simulink model "Single_Phase_grid-connected-inverter_Droop_inverter2"  (R2016b)
settings: Solver=VariableStepAuto  StartTime=0.0  StopTime=30  RelTol=1e-3
libraries: spsAlphaBetaZerotodq0Lib x4, simulink x4, spsSeriesRLCBranchLib x3, spsCurrentMeasurementLib x2, spsPWMGenerator2LevelLib x1, spsdq0toAlphaBetaZeroLib x1, spsDCVoltageSourceLib x1, spsPowerLib x1, spsUniversalBridgeLib x1, spsVoltageMeasurementLib x1, spspowerguiLib x1
settings Model: Creator=SALLEY  LastModifiedBy=49916
settings SimscapeCC: SimscapeNormalizeSystem=off

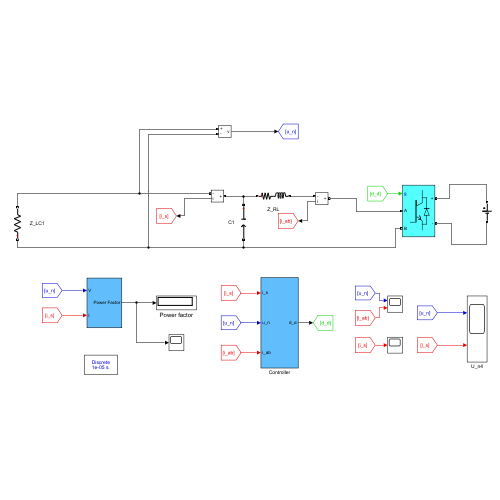
[thumbnail: Simulink's stored preview of the top-level diagram]
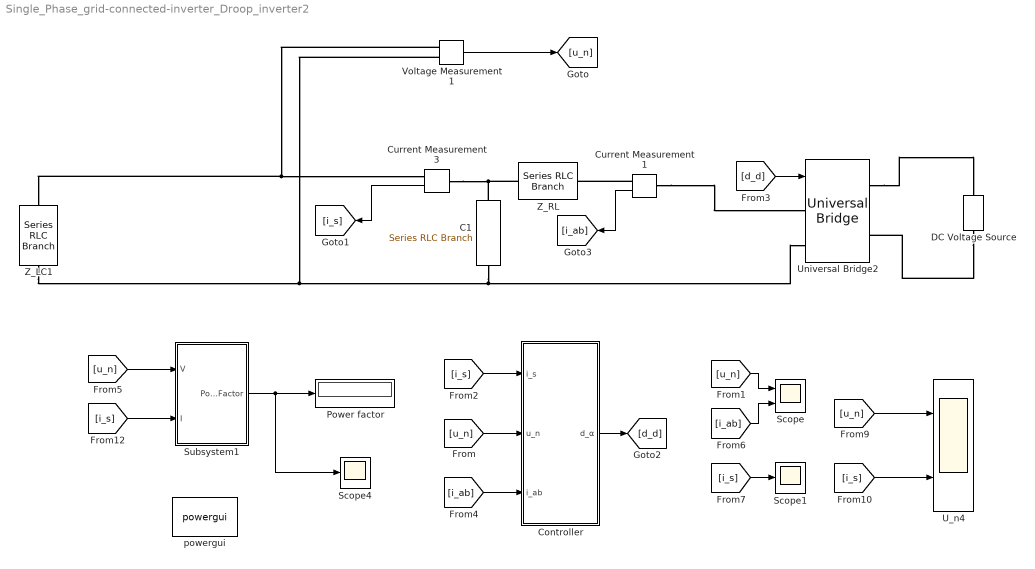
== system Single_Phase_grid-connected-inverter_Droop_inverter2 ==
  C1 : spsSeriesRLCBranchLib/Series RLC Branch  LConnTagsString=__new0  RConnTagsString=__new0  BranchType=C  Resistance=1  Inductance=1e-3  SetiL0=off  InitialCurrent=0  Capacitance=2e-5  Setx0=off  InitialVoltage=1500  Measurements=None
  Controller : Subsystem
  Current Measurement1 : spsCurrentMeasurementLib/Current Measurement  PhasorSimulation=off  OutputType=Complex  PSBequivalent=0
  Current Measurement3 : spsCurrentMeasurementLib/Current Measurement  PhasorSimulation=off  OutputType=Complex  PSBequivalent=0
  DC Voltage Source : spsDCVoltageSourceLib/DC Voltage Source  Amplitude=800  Measurements=None
  Power factor : Display
  Scope : Scope  NumInputPorts=2
  Scope1 : Scope
  Scope4 : Scope
  Subsystem1 : Subsystem
  U_n4 : Scope  NumInputPorts=2
  Universal Bridge2 : spsUniversalBridgeLib/Universal Bridge  Arms=2  SnubberResistance=1e5  SnubberCapacitance=inf  Device=IGBT / Diodes  Ron=1e-3  Lon=0  ForwardVoltages="[  0  0  ]"  ForwardVoltage=0  GTOparameters=[ 10e-6 , 20e-6 ]  IGBTparameters=[ 1e-6 , 2e-6 ]  Measurements=None  Measurements_2=None  converterType=Rectifier
  Voltage Measurement1 : spsVoltageMeasurementLib/Voltage Measurement  PhasorSimulation=off  OutputType=Complex  PSBequivalent=0
  Z_LC1 : spsSeriesRLCBranchLib/Series RLC Branch  LConnTagsString=__new0  RConnTagsString=__new0  BranchType=R  Resistance=2  Inductance=0  SetiL0=off  InitialCurrent=400  Capacitance=9.85e-3  Setx0=off  InitialVoltage=0  Measurements=None
  Z_RL : spsSeriesRLCBranchLib/Series RLC Branch  LConnTagsString=__new0  RConnTagsString=__new0  BranchType=RL  Resistance=0.2  Inductance=3e-3  SetiL0=off  InitialCurrent=400  Capacitance=9.85e-3  Setx0=off  InitialVoltage=0  Measurements=None
  powergui : spspowerguiLib/powergui  Priority=1  SimulationMode=Discrete  SampleTime=10e-6  frequency=60  Iterations=50  frequencyindice=0  Pbase=100e6  ErrMax=1e-4  UnitsV=kV  UnitsW=MW  buscounter=0  FunctionMessages=off  echomessages=off  EnableUseOfTLC=off  CurrentSourceSwitches=off  DisableSnubberDevices=off  DisableRonSwitches=off  DisableVfSwitches=off  DisplayEquations=off  AutomaticDiscreteSolvers=off  SolverType=Tustin/Backward Euler (TBE)  Interpol=off  ExternalGateDelay=off  methode=off  Ts=10  x0status=blocks  SPID=off  SwTol=0  HookPort=off  NonlinearTolerance=1e-4  nMaxIteration=100  ContinueOnMaxIteration=off  RestoreLinks=warning  ResistiveCurrentMeasurement=off  Frange=[0:2:500]  Ylog=off  Xlog=on  ShowGrid=off  save=off  variable=ZData  structure=0  ZoomFFT=off  StartTime=0.0  cycles=1  DisplayStyle=1  fundamental=60  FreqAxis=off  MaxFrequency=1000  frequencyindicesteady=1  RmsSteady=1  display=off
  wires:
  Current Measurement3/1 -> [i_s]
  Voltage Measurement1/1 -> [u_n]
  [u_n] -> Controller/2(u_n)
  [i_s] -> Controller/1(i_s)
  Controller/1(d_α) -> [d_d]
  [d_d] -> Universal Bridge2/1
  [i_s] -> Scope1/1
  [i_s] -> U_n4/2
  [u_n] -> Subsystem1/1(V)
  [i_s] -> Subsystem1/2(I)
  Subsystem1/1(Power Factor) -> Scope4/1, Power factor/1
  [u_n] -> Scope/1
  [u_n] -> U_n4/1
  [i_ab] -> Controller/3(i_ab)
  [i_ab] -> Scope/2
  Current Measurement1/1 -> [i_ab]
  connections:
  DC Voltage Source/LConn1 -- Universal Bridge2/RConn2
  Voltage Measurement1/LConn2 -- Z_LC1/LConn1 -- Universal Bridge2/LConn2 -- C1/RConn1
  Z_RL/LConn1 -- Current Measurement3/LConn1 -- C1/LConn1
  Voltage Measurement1/LConn1 -- Current Measurement3/RConn1 -- Z_LC1/RConn1
  Universal Bridge2/RConn1 -- DC Voltage Source/RConn1
  Current Measurement1/RConn1 -- Z_RL/RConn1
  Current Measurement1/LConn1 -- Universal Bridge2/LConn1

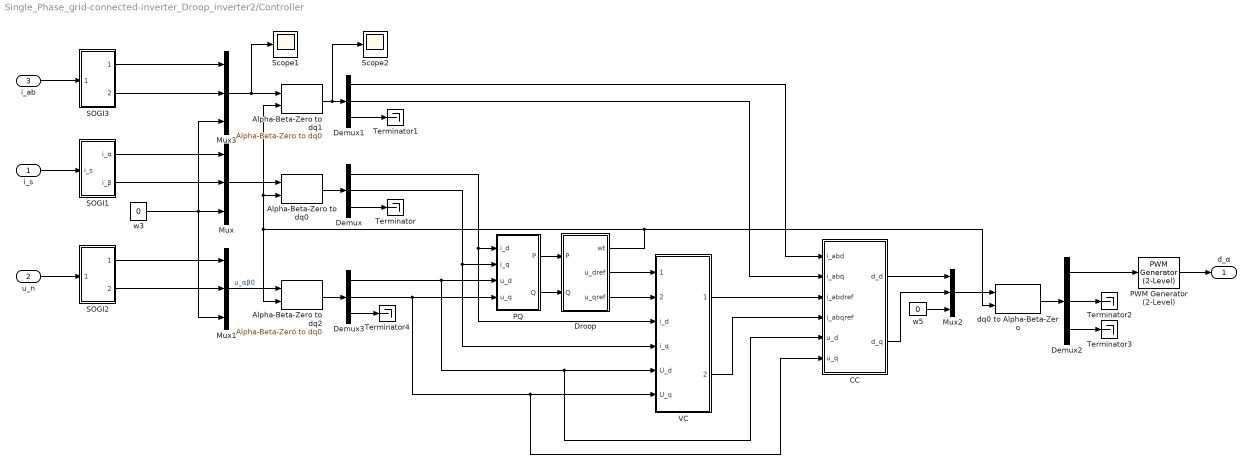
== system Single_Phase_grid-connected-inverter_Droop_inverter2/Controller ==
  i_s : Inport
  u_n : Inport  Port=2
  i_ab : Inport  Port=3
  Alpha-Beta-Zero to dq0 : spsAlphaBetaZerotodq0Lib/Alpha-Beta-Zero to dq0  Alignment=Aligned with phase A axis
  Alpha-Beta-Zero to dq1 : spsAlphaBetaZerotodq0Lib/Alpha-Beta-Zero to dq0  Alignment=Aligned with phase A axis
  Alpha-Beta-Zero to dq2 : spsAlphaBetaZerotodq0Lib/Alpha-Beta-Zero to dq0  Alignment=Aligned with phase A axis
  CC : Subsystem
  Demux{,1..3} (4 alike) : Demux  Outputs=3
  Droop : Subsystem
  Mux{,1..3} (4 alike) : Mux  Inputs=3
  PQ : Subsystem
  PWM Generator (2-Level) : spsPWMGenerator2LevelLib/PWM Generator (2-Level)  ModulatorType=Single-phase full-bridge (4 pulses)  ModulatorMode=Unsynchronized  Fc=1250  Pc=0  nF=27  MinMax="[ -1  1 ]"  SamplingTechnique=Natural  ModulatingSignals=off  m=0.8  Freq=60  Phase=0  Ts=2e-6  ShowCarrierOutport=off
  SOGI1 : Subsystem
  SOGI2 : Subsystem
  SOGI3 : Subsystem
  Scope1 : Scope
  Scope2 : Scope
  Terminator{,1..4} (5 alike) : Terminator
  VC : Subsystem
  dq0 to Alpha-Beta-Zero : spsdq0toAlphaBetaZeroLib/dq0 to Alpha-Beta-Zero  Alignment=Aligned with phase A axis
  w3 : Constant  Value=0
  w5 : Constant  Value=0
  d_α : Outport
  wires:
  Alpha-Beta-Zero to dq0/1 -> Demux/1
  Mux2/1 -> dq0 to Alpha-Beta-Zero/1
  dq0 to Alpha-Beta-Zero/1 -> Demux2/1
  Demux/3 -> Terminator/1
  Demux2/2 -> Terminator2/1
  Demux2/3 -> Terminator3/1
  Mux/1 -> Alpha-Beta-Zero to dq0/1
  w3/1 -> Mux1/3, Mux3/3, Mux/3
  w5/1 -> Mux2/3
  i_s/1 -> SOGI1/1(i_s)
  SOGI1/1(i_α) -> Mux/1
  SOGI1/2(i_β) -> Mux/2
  u_n/1 -> SOGI2/1(u_n)
  SOGI2/1(u_α) -> Mux1/1
  SOGI2/2(u_β) -> Mux1/2
  Mux1/1 -> Alpha-Beta-Zero to dq2/1  "u_αβ0"
  Demux3/1 -> CC/5(u_d), VC/5(U_d), PQ/3(u_d)
  Demux3/2 -> CC/6(u_q), VC/6(U_q), PQ/4(u_q)
  CC/1(d_d) -> Mux2/1
  CC/2(d_q) -> Mux2/2
  VC/1(i_abdref) -> CC/3(i_abdref)
  VC/2(i_abqref) -> CC/4(i_abqref)
  Droop/3(u_qref) -> VC/2(U_qref)
  i_ab/1 -> SOGI3/1(i_ab)
  SOGI3/1(i_abα) -> Mux3/1
  SOGI3/2(i_abβ) -> Mux3/2
  Mux3/1 -> Scope1/1, Alpha-Beta-Zero to dq1/1
  Alpha-Beta-Zero to dq1/1 -> Scope2/1, Demux1/1
  Demux1/3 -> Terminator1/1
  Demux1/1 -> CC/1(i_abd)
  Demux1/2 -> CC/2(i_abq)
  Demux/2 -> VC/4(i_q), PQ/2(i_q)
  Demux/1 -> VC/3(i_d), PQ/1(i_d)
  Alpha-Beta-Zero to dq2/1 -> Demux3/1
  Demux3/3 -> Terminator4/1
  PQ/1(P) -> Droop/1(P)
  PQ/2(Q) -> Droop/2(Q)
  Droop/1(wt) -> Alpha-Beta-Zero to dq2/2, Alpha-Beta-Zero to dq1/2, Alpha-Beta-Zero to dq0/2, dq0 to Alpha-Beta-Zero/2
  Droop/2(u_dref) -> VC/1(U_dref)
  Demux2/1 -> PWM Generator (2-Level)/1
  PWM Generator (2-Level)/1 -> d_α/1

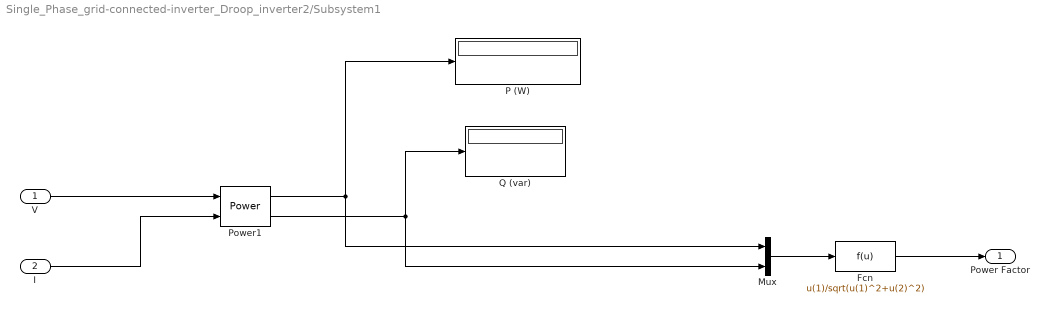
== system Single_Phase_grid-connected-inverter_Droop_inverter2/Subsystem1 ==
  V : Inport
  I : Inport  Port=2
  Fcn : Fcn  Expr=u(1)/sqrt(u(1)^2+u(2)^2)
  Mux : Mux  Inputs=2
  P (W) : Display
  Power1 : spsPowerLib/Power  Freq=50  Vinit=[1550*sqrt(2) 0]  Iinit=[15*sqrt(2) -15]  Ts=0
  Q (var) : Display
  Power Factor : Outport
  wires:
  Power1/2 -> Mux/2, Q (var)/1
  I/1 -> Power1/2
  Fcn/1 -> Power Factor/1
  Mux/1 -> Fcn/1
  V/1 -> Power1/1
  Power1/1 -> P (W)/1, Mux/1

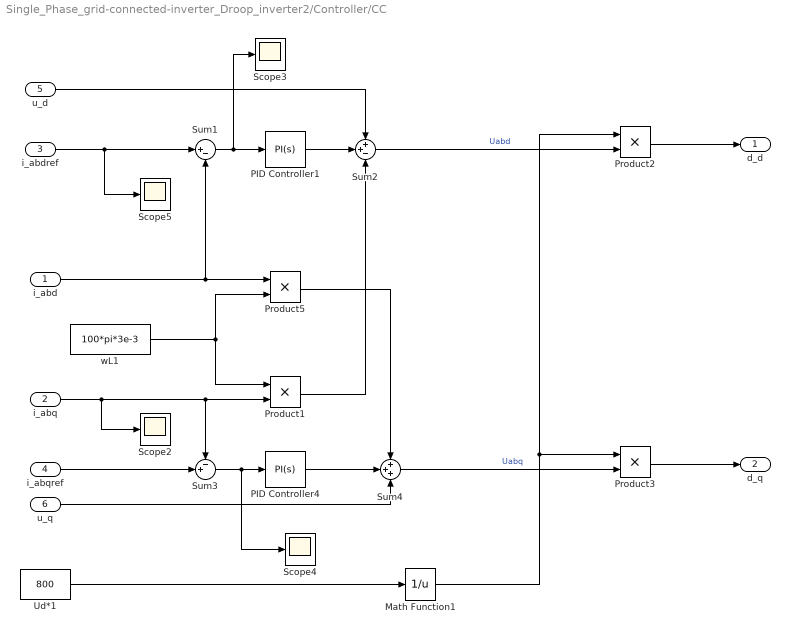
== system Single_Phase_grid-connected-inverter_Droop_inverter2/Controller/CC ==
  i_abd : Inport
  i_abq : Inport  Port=2
  i_abdref : Inport  Port=3
  i_abqref : Inport  Port=4
  u_d : Inport  Port=5
  u_q : Inport  Port=6
  Math Function1 : Math  Operator=reciprocal  SaturateOnIntegerOverflow=on
  PID Controller1 : simulink/Continuous/PID Controller  Controller=PI  Form=Parallel  TimeDomain=Continuous-time  SampleTime=-1  IntegratorMethod=Forward Euler  ControllerParametersSource=internal  P=50  I=100  D=0  UseFilter=on  N=100  InitialConditionSource=internal  InitialConditionForIntegrator=0  InitialConditionForFilter=0  DifferentiatorICPrevScaledInput=0  ExternalReset=none  TrackingMode=off  Kt=1  LimitOutput=off  UpperSaturationLimit=inf  LowerSaturationLimit=-inf  LinearizeAsGain=on  AntiWindupMode=none  Kb=1  POutMin=[]  POutMax=[]  IOutMin=[]  IOutMax=[]  DOutMin=[]  DOutMax=[]  NOutMin=[]  NOutMax=[]  SumOutMin=[]  SumOutMax=[]  SaturationOutMin=[]  SaturationOutMax=[]  PParamMin=[]  PParamMax=[]  IParamMin=[]  IParamMax=[]  DParamMin=[]  DParamMax=[]  NParamMin=[]  NParamMax=[]  KbParamMin=[]  KbParamMax=[]  KtParamMin=[]  KtParamMax=[]  KbOutMin=[]  KbOutMax=[]  KtOutMin=[]  KtOutMax=[]  IntegratorOutMin=[]  IntegratorOutMax=[]  FilterOutMin=[]  FilterOutMax=[]  SumI1OutMin=[]  SumI1OutMax=[]  SumI2OutMin=[]  SumI2OutMax=[]  SumI3OutMin=[]  SumI3OutMax=[]  SumDOutMin=[]  SumDOutMax=[]  DifferentiatorOutMin=[]  DifferentiatorOutMax=[]  IntegratorContinuousStateAttributes=''  IntegratorStateMustResolveToSignalObject=off  IntegratorRTWStateStorageClass=Auto  FilterContinuousStateAttributes=''  FilterStateMustResolveToSignalObject=off  FilterRTWStateStorageClass=Auto
  PID Controller4 : simulink/Continuous/PID Controller  Controller=PI  Form=Parallel  TimeDomain=Continuous-time  SampleTime=-1  IntegratorMethod=Forward Euler  ControllerParametersSource=internal  P=50  I=100  D=0  UseFilter=on  N=100  InitialConditionSource=internal  InitialConditionForIntegrator=0  InitialConditionForFilter=0  DifferentiatorICPrevScaledInput=0  ExternalReset=none  TrackingMode=off  Kt=1  LimitOutput=off  UpperSaturationLimit=inf  LowerSaturationLimit=-inf  LinearizeAsGain=on  AntiWindupMode=none  Kb=1  POutMin=[]  POutMax=[]  IOutMin=[]  IOutMax=[]  DOutMin=[]  DOutMax=[]  NOutMin=[]  NOutMax=[]  SumOutMin=[]  SumOutMax=[]  SaturationOutMin=[]  SaturationOutMax=[]  PParamMin=[]  PParamMax=[]  IParamMin=[]  IParamMax=[]  DParamMin=[]  DParamMax=[]  NParamMin=[]  NParamMax=[]  KbParamMin=[]  KbParamMax=[]  KtParamMin=[]  KtParamMax=[]  KbOutMin=[]  KbOutMax=[]  KtOutMin=[]  KtOutMax=[]  IntegratorOutMin=[]  IntegratorOutMax=[]  FilterOutMin=[]  FilterOutMax=[]  SumI1OutMin=[]  SumI1OutMax=[]  SumI2OutMin=[]  SumI2OutMax=[]  SumI3OutMin=[]  SumI3OutMax=[]  SumDOutMin=[]  SumDOutMax=[]  DifferentiatorOutMin=[]  DifferentiatorOutMax=[]  IntegratorContinuousStateAttributes=''  IntegratorStateMustResolveToSignalObject=off  IntegratorRTWStateStorageClass=Auto  FilterContinuousStateAttributes=''  FilterStateMustResolveToSignalObject=off  FilterRTWStateStorageClass=Auto
  Product{1..3,5} (4 alike) : Product
  Scope{2..5} (4 alike) : Scope
  Sum1 : Sum  Inputs=|+-
  Sum2 : Sum  Inputs=++-
  Sum3 : Sum  Inputs=-+|
  Sum4 : Sum  Inputs=+++
  Ud*1 : Constant  Value=800
  wL1 : Constant  Value=100*pi*3e-3
  d_d : Outport
  d_q : Outport  Port=2
  wires:
  PID Controller4/1 -> Sum4/2
  Product1/1 -> Sum2/3
  PID Controller1/1 -> Sum2/2
  wL1/1 -> Product5/2, Product1/1
  i_abqref/1 -> Sum3/2
  Sum1/1 -> Scope3/1, PID Controller1/1
  i_abdref/1 -> Scope5/1, Sum1/1
  u_q/1 -> Sum4/3
  i_abd/1 -> Product5/1, Sum1/2
  Sum2/1 -> Product2/2  "Uabd"
  Product5/1 -> Sum4/1
  u_d/1 -> Sum2/1
  i_abq/1 -> Scope2/1, Product1/2, Sum3/1
  Sum4/1 -> Product3/2  "Uabq"
  Product2/1 -> d_d/1
  Product3/1 -> d_q/1
  Sum3/1 -> Scope4/1, PID Controller4/1
  Math Function1/1 -> Product2/1, Product3/1
  Ud*1/1 -> Math Function1/1

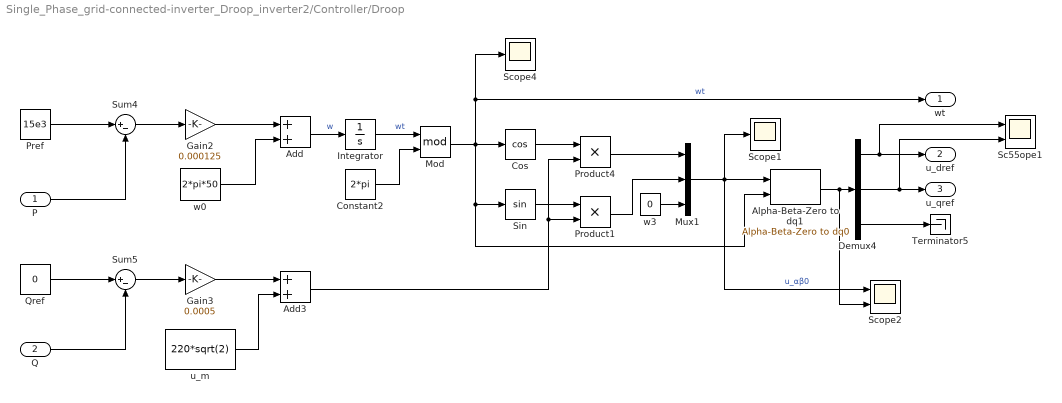
== system Single_Phase_grid-connected-inverter_Droop_inverter2/Controller/Droop ==
  P : Inport
  Q : Inport  Port=2
  Add : Sum
  Add3 : Sum
  Alpha-Beta-Zero to dq1 : spsAlphaBetaZerotodq0Lib/Alpha-Beta-Zero to dq0  Alignment=Aligned with phase A axis
  Constant2 : Constant  Value=2*pi
  Cos : Trigonometry  Operator=cos
  Demux4 : Demux  Outputs=3
  Gain2 : Gain  Gain=0.000125
  Gain3 : Gain  Gain=0.0005
  Integrator : Integrator
  Mod : Math  Operator=mod  SaturateOnIntegerOverflow=on
  Mux1 : Mux  Inputs=3
  Pref : Constant  Value=15e3
  Product1 : Product
  Product4 : Product
  Qref : Constant  Value=0
  Sc55ope1 : Scope  NumInputPorts=2
  Scope1 : Scope
  Scope2 : Scope  NumInputPorts=2
  Scope4 : Scope
  Sin : Trigonometry
  Sum4 : Sum  Inputs=|+-
  Sum5 : Sum  Inputs=|+-
  Terminator5 : Terminator
  u_m : Constant  Value=220*sqrt(2)
  w0 : Constant  Value=2*pi*50
  w3 : Constant  Value=0
  wt : Outport
  u_dref : Outport  Port=2
  u_qref : Outport  Port=3
  wires:
  Cos/1 -> Product4/1
  Mod/1 -> Cos/1, Sin/1, Alpha-Beta-Zero to dq1/2, wt/1, Scope4/1  "wt"
  Sum4/1 -> Gain2/1
  Integrator/1 -> Mod/1  "wt"
  Demux4/2 -> Sc55ope1/2, u_qref/1
  Alpha-Beta-Zero to dq1/1 -> Scope2/2, Demux4/1
  Constant2/1 -> Mod/2
  Demux4/3 -> Terminator5/1
  Add3/1 -> Product1/2, Product4/2
  Demux4/1 -> u_dref/1, Sc55ope1/1
  Q/1 -> Sum5/2
  Qref/1 -> Sum5/1
  u_m/1 -> Add3/2
  Gain2/1 -> Add/1
  Gain3/1 -> Add3/1
  Add/1 -> Integrator/1  "w"
  Sum5/1 -> Gain3/1
  w0/1 -> Add/2
  P/1 -> Sum4/2
  Pref/1 -> Sum4/1
  Product4/1 -> Mux1/1
  Mux1/1 -> Alpha-Beta-Zero to dq1/1, Scope1/1, Scope2/1  "u_αβ0"
  Sin/1 -> Product1/1
  Product1/1 -> Mux1/2
  w3/1 -> Mux1/3

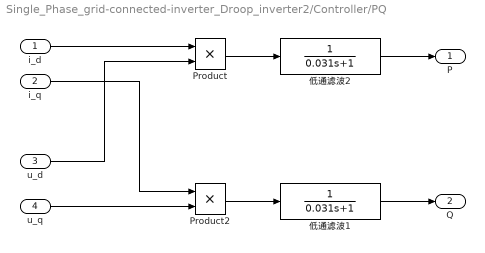
== system Single_Phase_grid-connected-inverter_Droop_inverter2/Controller/PQ ==
  i_d : Inport
  i_q : Inport  Port=2
  u_d : Inport  Port=3
  u_q : Inport  Port=4
  Product : Product
  Product2 : Product
  低通滤波1 : TransferFcn  Denominator=[0.031 1]
  低通滤波2 : TransferFcn  Denominator=[0.031 1]
  P : Outport
  Q : Outport  Port=2
  wires:
  Product/1 -> 低通滤波2/1
  低通滤波1/1 -> Q/1
  低通滤波2/1 -> P/1
  Product2/1 -> 低通滤波1/1
  i_d/1 -> Product/1
  i_q/1 -> Product2/1
  u_q/1 -> Product2/2
  u_d/1 -> Product/2

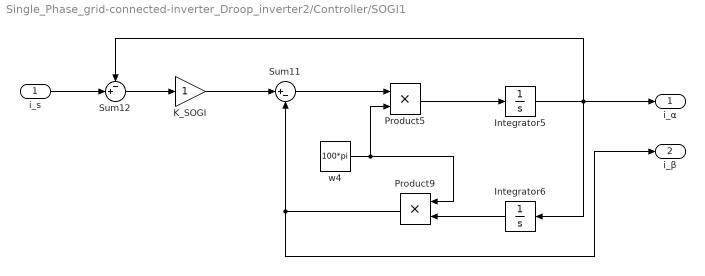
== system Single_Phase_grid-connected-inverter_Droop_inverter2/Controller/SOGI1 ==
  i_s : Inport
  Integrator5 : Integrator
  Integrator6 : Integrator
  K_SOGI : Gain
  Product5 : Product
  Product9 : Product
  Sum11 : Sum  Inputs=|+-
  Sum12 : Sum  Inputs=-+|
  w4 : Constant  Value=100*pi
  i_α : Outport
  i_β : Outport  Port=2
  wires:
  i_s/1 -> Sum12/2
  Integrator5/1 -> Sum12/1, i_α/1, Integrator6/1
  Product5/1 -> Integrator5/1
  Product9/1 -> i_β/1, Sum11/2
  w4/1 -> Product5/2, Product9/1
  Integrator6/1 -> Product9/2
  Sum12/1 -> K_SOGI/1
  Sum11/1 -> Product5/1
  K_SOGI/1 -> Sum11/1

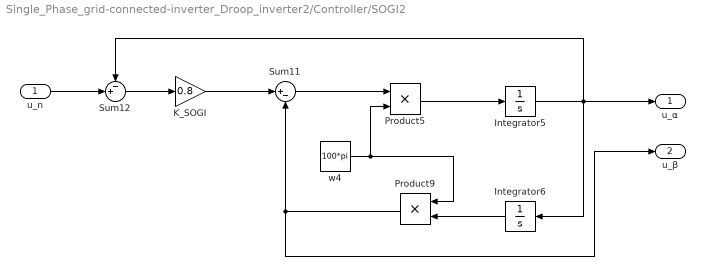
== system Single_Phase_grid-connected-inverter_Droop_inverter2/Controller/SOGI2 ==
  u_n : Inport
  Integrator5 : Integrator
  Integrator6 : Integrator
  K_SOGI : Gain  Gain=0.8
  Product5 : Product
  Product9 : Product
  Sum11 : Sum  Inputs=|+-
  Sum12 : Sum  Inputs=-+|
  w4 : Constant  Value=100*pi
  u_α : Outport
  u_β : Outport  Port=2
  wires:
  K_SOGI/1 -> Sum11/1
  Sum11/1 -> Product5/1
  Sum12/1 -> K_SOGI/1
  Integrator6/1 -> Product9/2
  w4/1 -> Product9/1, Product5/2
  Product9/1 -> Sum11/2, u_β/1
  Product5/1 -> Integrator5/1
  Integrator5/1 -> Integrator6/1, u_α/1, Sum12/1
  u_n/1 -> Sum12/2

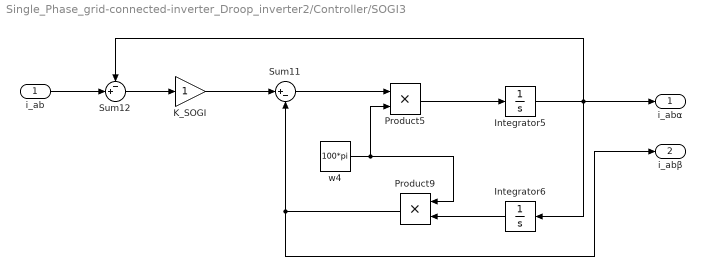
== system Single_Phase_grid-connected-inverter_Droop_inverter2/Controller/SOGI3 ==
  i_ab : Inport
  Integrator5 : Integrator
  Integrator6 : Integrator
  K_SOGI : Gain
  Product5 : Product
  Product9 : Product
  Sum11 : Sum  Inputs=|+-
  Sum12 : Sum  Inputs=-+|
  w4 : Constant  Value=100*pi
  i_abα : Outport
  i_abβ : Outport  Port=2
  wires:
  K_SOGI/1 -> Sum11/1
  Sum11/1 -> Product5/1
  Sum12/1 -> K_SOGI/1
  Integrator6/1 -> Product9/2
  w4/1 -> Product9/1, Product5/2
  Product9/1 -> Sum11/2, i_abβ/1
  Product5/1 -> Integrator5/1
  Integrator5/1 -> Integrator6/1, i_abα/1, Sum12/1
  i_ab/1 -> Sum12/2

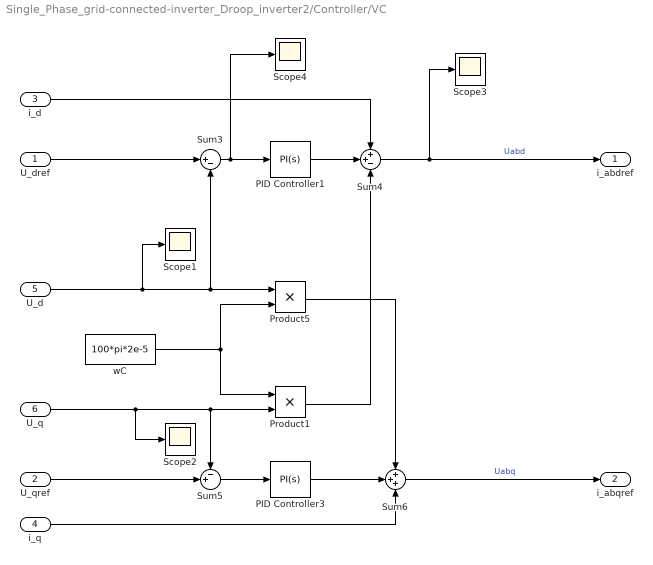
== system Single_Phase_grid-connected-inverter_Droop_inverter2/Controller/VC ==
  U_dref : Inport
  U_qref : Inport  Port=2
  i_d : Inport  Port=3
  i_q : Inport  Port=4
  U_d : Inport  Port=5
  U_q : Inport  Port=6
  PID Controller1 : simulink/Continuous/PID Controller  Controller=PI  Form=Parallel  TimeDomain=Continuous-time  SampleTime=-1  IntegratorMethod=Forward Euler  ControllerParametersSource=internal  P=0.3  I=10  D=0  UseFilter=on  N=100  InitialConditionSource=internal  InitialConditionForIntegrator=0  InitialConditionForFilter=0  DifferentiatorICPrevScaledInput=0  ExternalReset=none  TrackingMode=off  Kt=1  LimitOutput=off  UpperSaturationLimit=inf  LowerSaturationLimit=-inf  LinearizeAsGain=on  AntiWindupMode=none  Kb=1  POutMin=[]  POutMax=[]  IOutMin=[]  IOutMax=[]  DOutMin=[]  DOutMax=[]  NOutMin=[]  NOutMax=[]  SumOutMin=[]  SumOutMax=[]  SaturationOutMin=[]  SaturationOutMax=[]  PParamMin=[]  PParamMax=[]  IParamMin=[]  IParamMax=[]  DParamMin=[]  DParamMax=[]  NParamMin=[]  NParamMax=[]  KbParamMin=[]  KbParamMax=[]  KtParamMin=[]  KtParamMax=[]  KbOutMin=[]  KbOutMax=[]  KtOutMin=[]  KtOutMax=[]  IntegratorOutMin=[]  IntegratorOutMax=[]  FilterOutMin=[]  FilterOutMax=[]  SumI1OutMin=[]  SumI1OutMax=[]  SumI2OutMin=[]  SumI2OutMax=[]  SumI3OutMin=[]  SumI3OutMax=[]  SumDOutMin=[]  SumDOutMax=[]  DifferentiatorOutMin=[]  DifferentiatorOutMax=[]  IntegratorContinuousStateAttributes=''  IntegratorStateMustResolveToSignalObject=off  IntegratorRTWStateStorageClass=Auto  FilterContinuousStateAttributes=''  FilterStateMustResolveToSignalObject=off  FilterRTWStateStorageClass=Auto
  PID Controller3 : simulink/Continuous/PID Controller  Controller=PI  Form=Parallel  TimeDomain=Continuous-time  SampleTime=-1  IntegratorMethod=Forward Euler  ControllerParametersSource=internal  P=0.3  I=10  D=0  UseFilter=on  N=100  InitialConditionSource=internal  InitialConditionForIntegrator=0  InitialConditionForFilter=0  DifferentiatorICPrevScaledInput=0  ExternalReset=none  TrackingMode=off  Kt=1  LimitOutput=off  UpperSaturationLimit=inf  LowerSaturationLimit=-inf  LinearizeAsGain=on  AntiWindupMode=none  Kb=1  POutMin=[]  POutMax=[]  IOutMin=[]  IOutMax=[]  DOutMin=[]  DOutMax=[]  NOutMin=[]  NOutMax=[]  SumOutMin=[]  SumOutMax=[]  SaturationOutMin=[]  SaturationOutMax=[]  PParamMin=[]  PParamMax=[]  IParamMin=[]  IParamMax=[]  DParamMin=[]  DParamMax=[]  NParamMin=[]  NParamMax=[]  KbParamMin=[]  KbParamMax=[]  KtParamMin=[]  KtParamMax=[]  KbOutMin=[]  KbOutMax=[]  KtOutMin=[]  KtOutMax=[]  IntegratorOutMin=[]  IntegratorOutMax=[]  FilterOutMin=[]  FilterOutMax=[]  SumI1OutMin=[]  SumI1OutMax=[]  SumI2OutMin=[]  SumI2OutMax=[]  SumI3OutMin=[]  SumI3OutMax=[]  SumDOutMin=[]  SumDOutMax=[]  DifferentiatorOutMin=[]  DifferentiatorOutMax=[]  IntegratorContinuousStateAttributes=''  IntegratorStateMustResolveToSignalObject=off  IntegratorRTWStateStorageClass=Auto  FilterContinuousStateAttributes=''  FilterStateMustResolveToSignalObject=off  FilterRTWStateStorageClass=Auto
  Product1 : Product
  Product5 : Product
  Scope{1..4} (4 alike) : Scope
  Sum3 : Sum  Inputs=|+-
  Sum4 : Sum  Inputs=++-
  Sum5 : Sum  Inputs=-+|
  Sum6 : Sum  Inputs=+++
  wC : Constant  Value=100*pi*2e-5
  i_abdref : Outport
  i_abqref : Outport  Port=2
  wires:
  PID Controller3/1 -> Sum6/2
  Product1/1 -> Sum4/3
  PID Controller1/1 -> Sum4/2
  wC/1 -> Product5/2, Product1/1
  U_qref/1 -> Sum5/2
  Sum3/1 -> PID Controller1/1, Scope4/1
  U_dref/1 -> Sum3/1
  i_q/1 -> Sum6/3
  U_d/1 -> Product5/1, Sum3/2, Scope1/1
  Sum4/1 -> Scope3/1, i_abdref/1  "Uabd"
  Product5/1 -> Sum6/1
  i_d/1 -> Sum4/1
  U_q/1 -> Scope2/1, Product1/2, Sum5/1
  Sum6/1 -> i_abqref/1  "Uabq"
  Sum5/1 -> PID Controller3/1
